simulink model "AUV_MechanicsHullCAD"  (R2020a)
(part 3 of 12)

      mask help: This block creates a flat, single, square tile element. The square tile body is mass-less, so it will not have an effect on the dynamic simulation. This square tile element can be used as a graphic reference by itself, or as part of a composite graphic reference made of an array of interconnected tiles. The square tile is aligned with the XY plane, and the block provides frame connector ports to the middle points on each of the four sides of the body of the square - right (+X), left (-X), top (+Y) and bottom (-Y). All dimensions are in meters.
      settings: PortSchema="{\"entries\":[{\"content\":{\"sides\":[{\"content\":{\"connectorIds\":[\"LConn1\"]},\"type\":\"ConnectorPlacement.EquallySpacedRectSide\",\"uuid\":\"a971723f-ea37-4e9b-910b-501b94fb0ba2\"},{\"content\":{\"connectorIds\":[\"RConn1\"],\"side\":\"RIGHT\"},\"type\":\"ConnectorPlacement.EquallySpacedRectSide\",\"uuid\":\"e50175c1-005c-4b0b-bced-b882197eaab2\"},{\"content\":{\"connectorIds\":[\"LConn2\"],\"side\":\"TOP\"},\"type\":\"ConnectorPlacement.EquallySpacedRectSide\",\"uuid\":\"2a04a964-d53e-47ee-8c79-d53dd599bafe\"},{\"content\":{\"connectorIds\":[\"RConn2\"],\"side\":\"BOTTOM\"},\"type\":\"ConnectorPlacement.EquallySpacedRectSide\",\"uuid\":\"a0066dd6-a193-491c-afbe-bac00dfc3505\"}]},\"type\":\"ConnectorPlacement.EquallySpacedConnector\",\"uuid\":\"c80211c6-bb24-481b-97ca-2752015f3b18\"}],\"packageUris\":[\"http://schema.mathworks.com/mf0/Connector/19700101\"],\"version\":\"1.0\"}"
  Tile83 : Subsystem  mask(Square Tile){side=side, thickness=thick, color=color1, opacity=opacity}
      mask prompts: side "Side (m) :"; thickness "Thickness (m) :"; color "Color [RGB] :"; opacity "Opacity (0...1) :"
      mask help: This block creates a flat, single, square tile element. The square tile body is mass-less, so it will not have an effect on the dynamic simulation. This square tile element can be used as a graphic reference by itself, or as part of a composite graphic reference made of an array of interconnected tiles. The square tile is aligned with the XY plane, and the block provides frame connector ports to the middle points on each of the four sides of the body of the square - right (+X), left (-X), top (+Y) and bottom (-Y). All dimensions are in meters.
      settings: PortSchema="{\"entries\":[{\"content\":{\"sides\":[{\"content\":{\"connectorIds\":[\"LConn1\"]},\"type\":\"ConnectorPlacement.EquallySpacedRectSide\",\"uuid\":\"a971723f-ea37-4e9b-910b-501b94fb0ba2\"},{\"content\":{\"connectorIds\":[\"RConn1\"],\"side\":\"RIGHT\"},\"type\":\"ConnectorPlacement.EquallySpacedRectSide\",\"uuid\":\"e50175c1-005c-4b0b-bced-b882197eaab2\"},{\"content\":{\"connectorIds\":[\"LConn2\"],\"side\":\"TOP\"},\"type\":\"ConnectorPlacement.EquallySpacedRectSide\",\"uuid\":\"2a04a964-d53e-47ee-8c79-d53dd599bafe\"},{\"content\":{\"connectorIds\":[\"RConn2\"],\"side\":\"BOTTOM\"},\"type\":\"ConnectorPlacement.EquallySpacedRectSide\",\"uuid\":\"a0066dd6-a193-491c-afbe-bac00dfc3505\"}]},\"type\":\"ConnectorPlacement.EquallySpacedConnector\",\"uuid\":\"c80211c6-bb24-481b-97ca-2752015f3b18\"}],\"packageUris\":[\"http://schema.mathworks.com/mf0/Connector/19700101\"],\"version\":\"1.0\"}"
  Tile84 : Subsystem  mask(Square Tile){side=side, thickness=thick, color=color1, opacity=opacity}
      mask prompts: side "Side (m) :"; thickness "Thickness (m) :"; color "Color [RGB] :"; opacity "Opacity (0...1) :"
      mask help: This block creates a flat, single, square tile element. The square tile body is mass-less, so it will not have an effect on the dynamic simulation. This square tile element can be used as a graphic reference by itself, or as part of a composite graphic reference made of an array of interconnected tiles. The square tile is aligned with the XY plane, and the block provides frame connector ports to the middle points on each of the four sides of the body of the square - right (+X), left (-X), top (+Y) and bottom (-Y). All dimensions are in meters.
      settings: PortSchema="{\"entries\":[{\"content\":{\"sides\":[{\"content\":{\"connectorIds\":[\"LConn1\"]},\"type\":\"ConnectorPlacement.EquallySpacedRectSide\",\"uuid\":\"a971723f-ea37-4e9b-910b-501b94fb0ba2\"},{\"content\":{\"connectorIds\":[\"RConn1\"],\"side\":\"RIGHT\"},\"type\":\"ConnectorPlacement.EquallySpacedRectSide\",\"uuid\":\"e50175c1-005c-4b0b-bced-b882197eaab2\"},{\"content\":{\"connectorIds\":[\"LConn2\"],\"side\":\"TOP\"},\"type\":\"ConnectorPlacement.EquallySpacedRectSide\",\"uuid\":\"2a04a964-d53e-47ee-8c79-d53dd599bafe\"},{\"content\":{\"connectorIds\":[\"RConn2\"],\"side\":\"BOTTOM\"},\"type\":\"ConnectorPlacement.EquallySpacedRectSide\",\"uuid\":\"a0066dd6-a193-491c-afbe-bac00dfc3505\"}]},\"type\":\"ConnectorPlacement.EquallySpacedConnector\",\"uuid\":\"c80211c6-bb24-481b-97ca-2752015f3b18\"}],\"packageUris\":[\"http://schema.mathworks.com/mf0/Connector/19700101\"],\"version\":\"1.0\"}"
  Tile85 : Subsystem  mask(Square Tile){side=side, thickness=thick, color=color2, opacity=opacity}
      mask prompts: side "Side (m) :"; thickness "Thickness (m) :"; color "Color [RGB] :"; opacity "Opacity (0...1) :"
      mask help: This block creates a flat, single, square tile element. The square tile body is mass-less, so it will not have an effect on the dynamic simulation. This square tile element can be used as a graphic reference by itself, or as part of a composite graphic reference made of an array of interconnected tiles. The square tile is aligned with the XY plane, and the block provides frame connector ports to the middle points on each of the four sides of the body of the square - right (+X), left (-X), top (+Y) and bottom (-Y). All dimensions are in meters.
      settings: PortSchema="{\"entries\":[{\"content\":{\"sides\":[{\"content\":{\"connectorIds\":[\"LConn1\"]},\"type\":\"ConnectorPlacement.EquallySpacedRectSide\",\"uuid\":\"a971723f-ea37-4e9b-910b-501b94fb0ba2\"},{\"content\":{\"connectorIds\":[\"RConn1\"],\"side\":\"RIGHT\"},\"type\":\"ConnectorPlacement.EquallySpacedRectSide\",\"uuid\":\"e50175c1-005c-4b0b-bced-b882197eaab2\"},{\"content\":{\"connectorIds\":[\"LConn2\"],\"side\":\"TOP\"},\"type\":\"ConnectorPlacement.EquallySpacedRectSide\",\"uuid\":\"2a04a964-d53e-47ee-8c79-d53dd599bafe\"},{\"content\":{\"connectorIds\":[\"RConn2\"],\"side\":\"BOTTOM\"},\"type\":\"ConnectorPlacement.EquallySpacedRectSide\",\"uuid\":\"a0066dd6-a193-491c-afbe-bac00dfc3505\"}]},\"type\":\"ConnectorPlacement.EquallySpacedConnector\",\"uuid\":\"c80211c6-bb24-481b-97ca-2752015f3b18\"}],\"packageUris\":[\"http://schema.mathworks.com/mf0/Connector/19700101\"],\"version\":\"1.0\"}"
  Tile86 : Subsystem  mask(Square Tile){side=side, thickness=thick, color=color1, opacity=opacity}
      mask prompts: side "Side (m) :"; thickness "Thickness (m) :"; color "Color [RGB] :"; opacity "Opacity (0...1) :"
      mask help: This block creates a flat, single, square tile element. The square tile body is mass-less, so it will not have an effect on the dynamic simulation. This square tile element can be used as a graphic reference by itself, or as part of a composite graphic reference made of an array of interconnected tiles. The square tile is aligned with the XY plane, and the block provides frame connector ports to the middle points on each of the four sides of the body of the square - right (+X), left (-X), top (+Y) and bottom (-Y). All dimensions are in meters.
      settings: PortSchema="{\"entries\":[{\"content\":{\"sides\":[{\"content\":{\"connectorIds\":[\"LConn1\"]},\"type\":\"ConnectorPlacement.EquallySpacedRectSide\",\"uuid\":\"a971723f-ea37-4e9b-910b-501b94fb0ba2\"},{\"content\":{\"connectorIds\":[\"RConn1\"],\"side\":\"RIGHT\"},\"type\":\"ConnectorPlacement.EquallySpacedRectSide\",\"uuid\":\"e50175c1-005c-4b0b-bced-b882197eaab2\"},{\"content\":{\"connectorIds\":[\"LConn2\"],\"side\":\"TOP\"},\"type\":\"ConnectorPlacement.EquallySpacedRectSide\",\"uuid\":\"2a04a964-d53e-47ee-8c79-d53dd599bafe\"},{\"content\":{\"connectorIds\":[\"RConn2\"],\"side\":\"BOTTOM\"},\"type\":\"ConnectorPlacement.EquallySpacedRectSide\",\"uuid\":\"a0066dd6-a193-491c-afbe-bac00dfc3505\"}]},\"type\":\"ConnectorPlacement.EquallySpacedConnector\",\"uuid\":\"c80211c6-bb24-481b-97ca-2752015f3b18\"}],\"packageUris\":[\"http://schema.mathworks.com/mf0/Connector/19700101\"],\"version\":\"1.0\"}"
  Tile87 : Subsystem  mask(Square Tile){side=side, thickness=thick, color=color2, opacity=opacity}
      mask prompts: side "Side (m) :"; thickness "Thickness (m) :"; color "Color [RGB] :"; opacity "Opacity (0...1) :"
      mask help: This block creates a flat, single, square tile element. The square tile body is mass-less, so it will not have an effect on the dynamic simulation. This square tile element can be used as a graphic reference by itself, or as part of a composite graphic reference made of an array of interconnected tiles. The square tile is aligned with the XY plane, and the block provides frame connector ports to the middle points on each of the four sides of the body of the square - right (+X), left (-X), top (+Y) and bottom (-Y). All dimensions are in meters.
      settings: PortSchema="{\"entries\":[{\"content\":{\"sides\":[{\"content\":{\"connectorIds\":[\"LConn1\"]},\"type\":\"ConnectorPlacement.EquallySpacedRectSide\",\"uuid\":\"a971723f-ea37-4e9b-910b-501b94fb0ba2\"},{\"content\":{\"connectorIds\":[\"RConn1\"],\"side\":\"RIGHT\"},\"type\":\"ConnectorPlacement.EquallySpacedRectSide\",\"uuid\":\"e50175c1-005c-4b0b-bced-b882197eaab2\"},{\"content\":{\"connectorIds\":[\"LConn2\"],\"side\":\"TOP\"},\"type\":\"ConnectorPlacement.EquallySpacedRectSide\",\"uuid\":\"2a04a964-d53e-47ee-8c79-d53dd599bafe\"},{\"content\":{\"connectorIds\":[\"RConn2\"],\"side\":\"BOTTOM\"},\"type\":\"ConnectorPlacement.EquallySpacedRectSide\",\"uuid\":\"a0066dd6-a193-491c-afbe-bac00dfc3505\"}]},\"type\":\"ConnectorPlacement.EquallySpacedConnector\",\"uuid\":\"c80211c6-bb24-481b-97ca-2752015f3b18\"}],\"packageUris\":[\"http://schema.mathworks.com/mf0/Connector/19700101\"],\"version\":\"1.0\"}"
  Tile88 : Subsystem  mask(Square Tile){side=side, thickness=thick, color=color1, opacity=opacity}
      mask prompts: side "Side (m) :"; thickness "Thickness (m) :"; color "Color [RGB] :"; opacity "Opacity (0...1) :"
      mask help: This block creates a flat, single, square tile element. The square tile body is mass-less, so it will not have an effect on the dynamic simulation. This square tile element can be used as a graphic reference by itself, or as part of a composite graphic reference made of an array of interconnected tiles. The square tile is aligned with the XY plane, and the block provides frame connector ports to the middle points on each of the four sides of the body of the square - right (+X), left (-X), top (+Y) and bottom (-Y). All dimensions are in meters.
      settings: PortSchema="{\"entries\":[{\"content\":{\"sides\":[{\"content\":{\"connectorIds\":[\"LConn1\"]},\"type\":\"ConnectorPlacement.EquallySpacedRectSide\",\"uuid\":\"a971723f-ea37-4e9b-910b-501b94fb0ba2\"},{\"content\":{\"connectorIds\":[\"RConn1\"],\"side\":\"RIGHT\"},\"type\":\"ConnectorPlacement.EquallySpacedRectSide\",\"uuid\":\"e50175c1-005c-4b0b-bced-b882197eaab2\"},{\"content\":{\"connectorIds\":[\"LConn2\"],\"side\":\"TOP\"},\"type\":\"ConnectorPlacement.EquallySpacedRectSide\",\"uuid\":\"2a04a964-d53e-47ee-8c79-d53dd599bafe\"},{\"content\":{\"connectorIds\":[\"RConn2\"],\"side\":\"BOTTOM\"},\"type\":\"ConnectorPlacement.EquallySpacedRectSide\",\"uuid\":\"a0066dd6-a193-491c-afbe-bac00dfc3505\"}]},\"type\":\"ConnectorPlacement.EquallySpacedConnector\",\"uuid\":\"c80211c6-bb24-481b-97ca-2752015f3b18\"}],\"packageUris\":[\"http://schema.mathworks.com/mf0/Connector/19700101\"],\"version\":\"1.0\"}"
  Tile89 : Subsystem  mask(Square Tile){side=side, thickness=thick, color=color2, opacity=opacity}
      mask prompts: side "Side (m) :"; thickness "Thickness (m) :"; color "Color [RGB] :"; opacity "Opacity (0...1) :"
      mask help: This block creates a flat, single, square tile element. The square tile body is mass-less, so it will not have an effect on the dynamic simulation. This square tile element can be used as a graphic reference by itself, or as part of a composite graphic reference made of an array of interconnected tiles. The square tile is aligned with the XY plane, and the block provides frame connector ports to the middle points on each of the four sides of the body of the square - right (+X), left (-X), top (+Y) and bottom (-Y). All dimensions are in meters.
      settings: PortSchema="{\"entries\":[{\"content\":{\"sides\":[{\"content\":{\"connectorIds\":[\"LConn1\"]},\"type\":\"ConnectorPlacement.EquallySpacedRectSide\",\"uuid\":\"a971723f-ea37-4e9b-910b-501b94fb0ba2\"},{\"content\":{\"connectorIds\":[\"RConn1\"],\"side\":\"RIGHT\"},\"type\":\"ConnectorPlacement.EquallySpacedRectSide\",\"uuid\":\"e50175c1-005c-4b0b-bced-b882197eaab2\"},{\"content\":{\"connectorIds\":[\"LConn2\"],\"side\":\"TOP\"},\"type\":\"ConnectorPlacement.EquallySpacedRectSide\",\"uuid\":\"2a04a964-d53e-47ee-8c79-d53dd599bafe\"},{\"content\":{\"connectorIds\":[\"RConn2\"],\"side\":\"BOTTOM\"},\"type\":\"ConnectorPlacement.EquallySpacedRectSide\",\"uuid\":\"a0066dd6-a193-491c-afbe-bac00dfc3505\"}]},\"type\":\"ConnectorPlacement.EquallySpacedConnector\",\"uuid\":\"c80211c6-bb24-481b-97ca-2752015f3b18\"}],\"packageUris\":[\"http://schema.mathworks.com/mf0/Connector/19700101\"],\"version\":\"1.0\"}"
  Tile9 : Subsystem  mask(Square Tile){side=side, thickness=thick, color=color1, opacity=opacity}
      mask prompts: side "Side (m) :"; thickness "Thickness (m) :"; color "Color [RGB] :"; opacity "Opacity (0...1) :"
      mask help: This block creates a flat, single, square tile element. The square tile body is mass-less, so it will not have an effect on the dynamic simulation. This square tile element can be used as a graphic reference by itself, or as part of a composite graphic reference made of an array of interconnected tiles. The square tile is aligned with the XY plane, and the block provides frame connector ports to the middle points on each of the four sides of the body of the square - right (+X), left (-X), top (+Y) and bottom (-Y). All dimensions are in meters.
      settings: PortSchema="{\"entries\":[{\"content\":{\"sides\":[{\"content\":{\"connectorIds\":[\"LConn1\"]},\"type\":\"ConnectorPlacement.EquallySpacedRectSide\",\"uuid\":\"a971723f-ea37-4e9b-910b-501b94fb0ba2\"},{\"content\":{\"connectorIds\":[\"RConn1\"],\"side\":\"RIGHT\"},\"type\":\"ConnectorPlacement.EquallySpacedRectSide\",\"uuid\":\"e50175c1-005c-4b0b-bced-b882197eaab2\"},{\"content\":{\"connectorIds\":[\"LConn2\"],\"side\":\"TOP\"},\"type\":\"ConnectorPlacement.EquallySpacedRectSide\",\"uuid\":\"2a04a964-d53e-47ee-8c79-d53dd599bafe\"},{\"content\":{\"connectorIds\":[\"RConn2\"],\"side\":\"BOTTOM\"},\"type\":\"ConnectorPlacement.EquallySpacedRectSide\",\"uuid\":\"a0066dd6-a193-491c-afbe-bac00dfc3505\"}]},\"type\":\"ConnectorPlacement.EquallySpacedConnector\",\"uuid\":\"c80211c6-bb24-481b-97ca-2752015f3b18\"}],\"packageUris\":[\"http://schema.mathworks.com/mf0/Connector/19700101\"],\"version\":\"1.0\"}"
  Tile90 : Subsystem  mask(Square Tile){side=side, thickness=thick, color=color1, opacity=opacity}
      mask prompts: side "Side (m) :"; thickness "Thickness (m) :"; color "Color [RGB] :"; opacity "Opacity (0...1) :"
      mask help: This block creates a flat, single, square tile element. The square tile body is mass-less, so it will not have an effect on the dynamic simulation. This square tile element can be used as a graphic reference by itself, or as part of a composite graphic reference made of an array of interconnected tiles. The square tile is aligned with the XY plane, and the block provides frame connector ports to the middle points on each of the four sides of the body of the square - right (+X), left (-X), top (+Y) and bottom (-Y). All dimensions are in meters.
      settings: PortSchema="{\"entries\":[{\"content\":{\"sides\":[{\"content\":{\"connectorIds\":[\"LConn1\"]},\"type\":\"ConnectorPlacement.EquallySpacedRectSide\",\"uuid\":\"a971723f-ea37-4e9b-910b-501b94fb0ba2\"},{\"content\":{\"connectorIds\":[\"RConn1\"],\"side\":\"RIGHT\"},\"type\":\"ConnectorPlacement.EquallySpacedRectSide\",\"uuid\":\"e50175c1-005c-4b0b-bced-b882197eaab2\"},{\"content\":{\"connectorIds\":[\"LConn2\"],\"side\":\"TOP\"},\"type\":\"ConnectorPlacement.EquallySpacedRectSide\",\"uuid\":\"2a04a964-d53e-47ee-8c79-d53dd599bafe\"},{\"content\":{\"connectorIds\":[\"RConn2\"],\"side\":\"BOTTOM\"},\"type\":\"ConnectorPlacement.EquallySpacedRectSide\",\"uuid\":\"a0066dd6-a193-491c-afbe-bac00dfc3505\"}]},\"type\":\"ConnectorPlacement.EquallySpacedConnector\",\"uuid\":\"c80211c6-bb24-481b-97ca-2752015f3b18\"}],\"packageUris\":[\"http://schema.mathworks.com/mf0/Connector/19700101\"],\"version\":\"1.0\"}"
  Tile91 : Subsystem  mask(Square Tile){side=side, thickness=thick, color=color1, opacity=opacity}
      mask prompts: side "Side (m) :"; thickness "Thickness (m) :"; color "Color [RGB] :"; opacity "Opacity (0...1) :"
      mask help: This block creates a flat, single, square tile element. The square tile body is mass-less, so it will not have an effect on the dynamic simulation. This square tile element can be used as a graphic reference by itself, or as part of a composite graphic reference made of an array of interconnected tiles. The square tile is aligned with the XY plane, and the block provides frame connector ports to the middle points on each of the four sides of the body of the square - right (+X), left (-X), top (+Y) and bottom (-Y). All dimensions are in meters.
      settings: PortSchema="{\"entries\":[{\"content\":{\"sides\":[{\"content\":{\"connectorIds\":[\"LConn1\"]},\"type\":\"ConnectorPlacement.EquallySpacedRectSide\",\"uuid\":\"a971723f-ea37-4e9b-910b-501b94fb0ba2\"},{\"content\":{\"connectorIds\":[\"RConn1\"],\"side\":\"RIGHT\"},\"type\":\"ConnectorPlacement.EquallySpacedRectSide\",\"uuid\":\"e50175c1-005c-4b0b-bced-b882197eaab2\"},{\"content\":{\"connectorIds\":[\"LConn2\"],\"side\":\"TOP\"},\"type\":\"ConnectorPlacement.EquallySpacedRectSide\",\"uuid\":\"2a04a964-d53e-47ee-8c79-d53dd599bafe\"},{\"content\":{\"connectorIds\":[\"RConn2\"],\"side\":\"BOTTOM\"},\"type\":\"ConnectorPlacement.EquallySpacedRectSide\",\"uuid\":\"a0066dd6-a193-491c-afbe-bac00dfc3505\"}]},\"type\":\"ConnectorPlacement.EquallySpacedConnector\",\"uuid\":\"c80211c6-bb24-481b-97ca-2752015f3b18\"}],\"packageUris\":[\"http://schema.mathworks.com/mf0/Connector/19700101\"],\"version\":\"1.0\"}"
  Tile92 : Subsystem  mask(Square Tile){side=side, thickness=thick, color=color2, opacity=opacity}
      mask prompts: side "Side (m) :"; thickness "Thickness (m) :"; color "Color [RGB] :"; opacity "Opacity (0...1) :"
      mask help: This block creates a flat, single, square tile element. The square tile body is mass-less, so it will not have an effect on the dynamic simulation. This square tile element can be used as a graphic reference by itself, or as part of a composite graphic reference made of an array of interconnected tiles. The square tile is aligned with the XY plane, and the block provides frame connector ports to the middle points on each of the four sides of the body of the square - right (+X), left (-X), top (+Y) and bottom (-Y). All dimensions are in meters.
      settings: PortSchema="{\"entries\":[{\"content\":{\"sides\":[{\"content\":{\"connectorIds\":[\"LConn1\"]},\"type\":\"ConnectorPlacement.EquallySpacedRectSide\",\"uuid\":\"a971723f-ea37-4e9b-910b-501b94fb0ba2\"},{\"content\":{\"connectorIds\":[\"RConn1\"],\"side\":\"RIGHT\"},\"type\":\"ConnectorPlacement.EquallySpacedRectSide\",\"uuid\":\"e50175c1-005c-4b0b-bced-b882197eaab2\"},{\"content\":{\"connectorIds\":[\"LConn2\"],\"side\":\"TOP\"},\"type\":\"ConnectorPlacement.EquallySpacedRectSide\",\"uuid\":\"2a04a964-d53e-47ee-8c79-d53dd599bafe\"},{\"content\":{\"connectorIds\":[\"RConn2\"],\"side\":\"BOTTOM\"},\"type\":\"ConnectorPlacement.EquallySpacedRectSide\",\"uuid\":\"a0066dd6-a193-491c-afbe-bac00dfc3505\"}]},\"type\":\"ConnectorPlacement.EquallySpacedConnector\",\"uuid\":\"c80211c6-bb24-481b-97ca-2752015f3b18\"}],\"packageUris\":[\"http://schema.mathworks.com/mf0/Connector/19700101\"],\"version\":\"1.0\"}"
  Tile93 : Subsystem  mask(Square Tile){side=side, thickness=thick, color=color2, opacity=opacity}
      mask prompts: side "Side (m) :"; thickness "Thickness (m) :"; color "Color [RGB] :"; opacity "Opacity (0...1) :"
      mask help: This block creates a flat, single, square tile element. The square tile body is mass-less, so it will not have an effect on the dynamic simulation. This square tile element can be used as a graphic reference by itself, or as part of a composite graphic reference made of an array of interconnected tiles. The square tile is aligned with the XY plane, and the block provides frame connector ports to the middle points on each of the four sides of the body of the square - right (+X), left (-X), top (+Y) and bottom (-Y). All dimensions are in meters.
      settings: PortSchema="{\"entries\":[{\"content\":{\"sides\":[{\"content\":{\"connectorIds\":[\"LConn1\"]},\"type\":\"ConnectorPlacement.EquallySpacedRectSide\",\"uuid\":\"a971723f-ea37-4e9b-910b-501b94fb0ba2\"},{\"content\":{\"connectorIds\":[\"RConn1\"],\"side\":\"RIGHT\"},\"type\":\"ConnectorPlacement.EquallySpacedRectSide\",\"uuid\":\"e50175c1-005c-4b0b-bced-b882197eaab2\"},{\"content\":{\"connectorIds\":[\"LConn2\"],\"side\":\"TOP\"},\"type\":\"ConnectorPlacement.EquallySpacedRectSide\",\"uuid\":\"2a04a964-d53e-47ee-8c79-d53dd599bafe\"},{\"content\":{\"connectorIds\":[\"RConn2\"],\"side\":\"BOTTOM\"},\"type\":\"ConnectorPlacement.EquallySpacedRectSide\",\"uuid\":\"a0066dd6-a193-491c-afbe-bac00dfc3505\"}]},\"type\":\"ConnectorPlacement.EquallySpacedConnector\",\"uuid\":\"c80211c6-bb24-481b-97ca-2752015f3b18\"}],\"packageUris\":[\"http://schema.mathworks.com/mf0/Connector/19700101\"],\"version\":\"1.0\"}"
  Tile94 : Subsystem  mask(Square Tile){side=side, thickness=thick, color=color1, opacity=opacity}
      mask prompts: side "Side (m) :"; thickness "Thickness (m) :"; color "Color [RGB] :"; opacity "Opacity (0...1) :"
      mask help: This block creates a flat, single, square tile element. The square tile body is mass-less, so it will not have an effect on the dynamic simulation. This square tile element can be used as a graphic reference by itself, or as part of a composite graphic reference made of an array of interconnected tiles. The square tile is aligned with the XY plane, and the block provides frame connector ports to the middle points on each of the four sides of the body of the square - right (+X), left (-X), top (+Y) and bottom (-Y). All dimensions are in meters.
      settings: PortSchema="{\"entries\":[{\"content\":{\"sides\":[{\"content\":{\"connectorIds\":[\"LConn1\"]},\"type\":\"ConnectorPlacement.EquallySpacedRectSide\",\"uuid\":\"a971723f-ea37-4e9b-910b-501b94fb0ba2\"},{\"content\":{\"connectorIds\":[\"RConn1\"],\"side\":\"RIGHT\"},\"type\":\"ConnectorPlacement.EquallySpacedRectSide\",\"uuid\":\"e50175c1-005c-4b0b-bced-b882197eaab2\"},{\"content\":{\"connectorIds\":[\"LConn2\"],\"side\":\"TOP\"},\"type\":\"ConnectorPlacement.EquallySpacedRectSide\",\"uuid\":\"2a04a964-d53e-47ee-8c79-d53dd599bafe\"},{\"content\":{\"connectorIds\":[\"RConn2\"],\"side\":\"BOTTOM\"},\"type\":\"ConnectorPlacement.EquallySpacedRectSide\",\"uuid\":\"a0066dd6-a193-491c-afbe-bac00dfc3505\"}]},\"type\":\"ConnectorPlacement.EquallySpacedConnector\",\"uuid\":\"c80211c6-bb24-481b-97ca-2752015f3b18\"}],\"packageUris\":[\"http://schema.mathworks.com/mf0/Connector/19700101\"],\"version\":\"1.0\"}"
  Tile95 : Subsystem  mask(Square Tile){side=side, thickness=thick, color=color2, opacity=opacity}
      mask prompts: side "Side (m) :"; thickness "Thickness (m) :"; color "Color [RGB] :"; opacity "Opacity (0...1) :"
      mask help: This block creates a flat, single, square tile element. The square tile body is mass-less, so it will not have an effect on the dynamic simulation. This square tile element can be used as a graphic reference by itself, or as part of a composite graphic reference made of an array of interconnected tiles. The square tile is aligned with the XY plane, and the block provides frame connector ports to the middle points on each of the four sides of the body of the square - right (+X), left (-X), top (+Y) and bottom (-Y). All dimensions are in meters.
      settings: PortSchema="{\"entries\":[{\"content\":{\"sides\":[{\"content\":{\"connectorIds\":[\"LConn1\"]},\"type\":\"ConnectorPlacement.EquallySpacedRectSide\",\"uuid\":\"a971723f-ea37-4e9b-910b-501b94fb0ba2\"},{\"content\":{\"connectorIds\":[\"RConn1\"],\"side\":\"RIGHT\"},\"type\":\"ConnectorPlacement.EquallySpacedRectSide\",\"uuid\":\"e50175c1-005c-4b0b-bced-b882197eaab2\"},{\"content\":{\"connectorIds\":[\"LConn2\"],\"side\":\"TOP\"},\"type\":\"ConnectorPlacement.EquallySpacedRectSide\",\"uuid\":\"2a04a964-d53e-47ee-8c79-d53dd599bafe\"},{\"content\":{\"connectorIds\":[\"RConn2\"],\"side\":\"BOTTOM\"},\"type\":\"ConnectorPlacement.EquallySpacedRectSide\",\"uuid\":\"a0066dd6-a193-491c-afbe-bac00dfc3505\"}]},\"type\":\"ConnectorPlacement.EquallySpacedConnector\",\"uuid\":\"c80211c6-bb24-481b-97ca-2752015f3b18\"}],\"packageUris\":[\"http://schema.mathworks.com/mf0/Connector/19700101\"],\"version\":\"1.0\"}"
  Tile96 : Subsystem  mask(Square Tile){side=side, thickness=thick, color=color1, opacity=opacity}
      mask prompts: side "Side (m) :"; thickness "Thickness (m) :"; color "Color [RGB] :"; opacity "Opacity (0...1) :"
      mask help: This block creates a flat, single, square tile element. The square tile body is mass-less, so it will not have an effect on the dynamic simulation. This square tile element can be used as a graphic reference by itself, or as part of a composite graphic reference made of an array of interconnected tiles. The square tile is aligned with the XY plane, and the block provides frame connector ports to the middle points on each of the four sides of the body of the square - right (+X), left (-X), top (+Y) and bottom (-Y). All dimensions are in meters.
      settings: PortSchema="{\"entries\":[{\"content\":{\"sides\":[{\"content\":{\"connectorIds\":[\"LConn1\"]},\"type\":\"ConnectorPlacement.EquallySpacedRectSide\",\"uuid\":\"a971723f-ea37-4e9b-910b-501b94fb0ba2\"},{\"content\":{\"connectorIds\":[\"RConn1\"],\"side\":\"RIGHT\"},\"type\":\"ConnectorPlacement.EquallySpacedRectSide\",\"uuid\":\"e50175c1-005c-4b0b-bced-b882197eaab2\"},{\"content\":{\"connectorIds\":[\"LConn2\"],\"side\":\"TOP\"},\"type\":\"ConnectorPlacement.EquallySpacedRectSide\",\"uuid\":\"2a04a964-d53e-47ee-8c79-d53dd599bafe\"},{\"content\":{\"connectorIds\":[\"RConn2\"],\"side\":\"BOTTOM\"},\"type\":\"ConnectorPlacement.EquallySpacedRectSide\",\"uuid\":\"a0066dd6-a193-491c-afbe-bac00dfc3505\"}]},\"type\":\"ConnectorPlacement.EquallySpacedConnector\",\"uuid\":\"c80211c6-bb24-481b-97ca-2752015f3b18\"}],\"packageUris\":[\"http://schema.mathworks.com/mf0/Connector/19700101\"],\"version\":\"1.0\"}"
  Tile97 : Subsystem  mask(Square Tile){side=side, thickness=thick, color=color2, opacity=opacity}
      mask prompts: side "Side (m) :"; thickness "Thickness (m) :"; color "Color [RGB] :"; opacity "Opacity (0...1) :"
      mask help: This block creates a flat, single, square tile element. The square tile body is mass-less, so it will not have an effect on the dynamic simulation. This square tile element can be used as a graphic reference by itself, or as part of a composite graphic reference made of an array of interconnected tiles. The square tile is aligned with the XY plane, and the block provides frame connector ports to the middle points on each of the four sides of the body of the square - right (+X), left (-X), top (+Y) and bottom (-Y). All dimensions are in meters.
      settings: PortSchema="{\"entries\":[{\"content\":{\"sides\":[{\"content\":{\"connectorIds\":[\"LConn1\"]},\"type\":\"ConnectorPlacement.EquallySpacedRectSide\",\"uuid\":\"a971723f-ea37-4e9b-910b-501b94fb0ba2\"},{\"content\":{\"connectorIds\":[\"RConn1\"],\"side\":\"RIGHT\"},\"type\":\"ConnectorPlacement.EquallySpacedRectSide\",\"uuid\":\"e50175c1-005c-4b0b-bced-b882197eaab2\"},{\"content\":{\"connectorIds\":[\"LConn2\"],\"side\":\"TOP\"},\"type\":\"ConnectorPlacement.EquallySpacedRectSide\",\"uuid\":\"2a04a964-d53e-47ee-8c79-d53dd599bafe\"},{\"content\":{\"connectorIds\":[\"RConn2\"],\"side\":\"BOTTOM\"},\"type\":\"ConnectorPlacement.EquallySpacedRectSide\",\"uuid\":\"a0066dd6-a193-491c-afbe-bac00dfc3505\"}]},\"type\":\"ConnectorPlacement.EquallySpacedConnector\",\"uuid\":\"c80211c6-bb24-481b-97ca-2752015f3b18\"}],\"packageUris\":[\"http://schema.mathworks.com/mf0/Connector/19700101\"],\"version\":\"1.0\"}"
  Tile98 : Subsystem  mask(Square Tile){side=side, thickness=thick, color=color1, opacity=opacity}
      mask prompts: side "Side (m) :"; thickness "Thickness (m) :"; color "Color [RGB] :"; opacity "Opacity (0...1) :"
      mask help: This block creates a flat, single, square tile element. The square tile body is mass-less, so it will not have an effect on the dynamic simulation. This square tile element can be used as a graphic reference by itself, or as part of a composite graphic reference made of an array of interconnected tiles. The square tile is aligned with the XY plane, and the block provides frame connector ports to the middle points on each of the four sides of the body of the square - right (+X), left (-X), top (+Y) and bottom (-Y). All dimensions are in meters.
      settings: PortSchema="{\"entries\":[{\"content\":{\"sides\":[{\"content\":{\"connectorIds\":[\"LConn1\"]},\"type\":\"ConnectorPlacement.EquallySpacedRectSide\",\"uuid\":\"a971723f-ea37-4e9b-910b-501b94fb0ba2\"},{\"content\":{\"connectorIds\":[\"RConn1\"],\"side\":\"RIGHT\"},\"type\":\"ConnectorPlacement.EquallySpacedRectSide\",\"uuid\":\"e50175c1-005c-4b0b-bced-b882197eaab2\"},{\"content\":{\"connectorIds\":[\"LConn2\"],\"side\":\"TOP\"},\"type\":\"ConnectorPlacement.EquallySpacedRectSide\",\"uuid\":\"2a04a964-d53e-47ee-8c79-d53dd599bafe\"},{\"content\":{\"connectorIds\":[\"RConn2\"],\"side\":\"BOTTOM\"},\"type\":\"ConnectorPlacement.EquallySpacedRectSide\",\"uuid\":\"a0066dd6-a193-491c-afbe-bac00dfc3505\"}]},\"type\":\"ConnectorPlacement.EquallySpacedConnector\",\"uuid\":\"c80211c6-bb24-481b-97ca-2752015f3b18\"}],\"packageUris\":[\"http://schema.mathworks.com/mf0/Connector/19700101\"],\"version\":\"1.0\"}"
  Tile99 : Subsystem  mask(Square Tile){side=side, thickness=thick, color=color2, opacity=opacity}
      mask prompts: side "Side (m) :"; thickness "Thickness (m) :"; color "Color [RGB] :"; opacity "Opacity (0...1) :"
      mask help: This block creates a flat, single, square tile element. The square tile body is mass-less, so it will not have an effect on the dynamic simulation. This square tile element can be used as a graphic reference by itself, or as part of a composite graphic reference made of an array of interconnected tiles. The square tile is aligned with the XY plane, and the block provides frame connector ports to the middle points on each of the four sides of the body of the square - right (+X), left (-X), top (+Y) and bottom (-Y). All dimensions are in meters.
      settings: PortSchema="{\"entries\":[{\"content\":{\"sides\":[{\"content\":{\"connectorIds\":[\"LConn1\"]},\"type\":\"ConnectorPlacement.EquallySpacedRectSide\",\"uuid\":\"a971723f-ea37-4e9b-910b-501b94fb0ba2\"},{\"content\":{\"connectorIds\":[\"RConn1\"],\"side\":\"RIGHT\"},\"type\":\"ConnectorPlacement.EquallySpacedRectSide\",\"uuid\":\"e50175c1-005c-4b0b-bced-b882197eaab2\"},{\"content\":{\"connectorIds\":[\"LConn2\"],\"side\":\"TOP\"},\"type\":\"ConnectorPlacement.EquallySpacedRectSide\",\"uuid\":\"2a04a964-d53e-47ee-8c79-d53dd599bafe\"},{\"content\":{\"connectorIds\":[\"RConn2\"],\"side\":\"BOTTOM\"},\"type\":\"ConnectorPlacement.EquallySpacedRectSide\",\"uuid\":\"a0066dd6-a193-491c-afbe-bac00dfc3505\"}]},\"type\":\"ConnectorPlacement.EquallySpacedConnector\",\"uuid\":\"c80211c6-bb24-481b-97ca-2752015f3b18\"}],\"packageUris\":[\"http://schema.mathworks.com/mf0/Connector/19700101\"],\"version\":\"1.0\"}"
  F : PMIOPort  Side=Left
  connections:
  F/RConn1 -- Tile1/LConn1
  Tile2/LConn1 -- Tile1/RConn1
  Tile4/LConn1 -- Tile3/RConn1
  Tile2/RConn1 -- Tile3/LConn1
  Tile6/RConn1 -- Tile7/LConn1
  Tile8/LConn1 -- Tile7/RConn1
  Tile6/LConn1 -- Tile5/RConn1
  Tile5/LConn1 -- Tile4/RConn1
  Tile10/LConn1 -- Tile9/RConn1
  Tile9/LConn1 -- Tile8/RConn1
  Tile15/LConn1 -- Tile14/RConn1
  Tile16/LConn1 -- Tile15/RConn1
  Tile16/RConn1 -- Tile17/LConn1
  Tile18/LConn1 -- Tile17/RConn1
  Tile11/LConn1 -- Tile19/RConn1
  Tile19/LConn1 -- Tile18/RConn1
  Tile12/RConn1 -- Tile13/LConn1
  Tile14/LConn1 -- Tile13/RConn1
  Tile12/LConn2 -- Tile1/RConn2
  Tile20/LConn1 -- Tile11/RConn1
  Tile24/LConn2 -- Tile21/RConn2
  Tile26/LConn1 -- Tile25/RConn1
  Tile24/RConn1 -- Tile25/LConn1
  Tile31/LConn1 -- Tile30/RConn1
  Tile30/LConn1 -- Tile29/RConn1
  Tile23/LConn1 -- Tile31/RConn1
  Tile28/RConn1 -- Tile29/LConn1
  Tile28/LConn1 -- Tile27/RConn1
  Tile27/LConn1 -- Tile26/RConn1
  Tile36/LConn1 -- Tile35/RConn1
  Tile37/LConn1 -- Tile36/RConn1
  Tile22/LConn1 -- Tile40/RConn1
  Tile37/RConn1 -- Tile38/LConn1
  Tile40/LConn1 -- Tile39/RConn1
  Tile39/LConn1 -- Tile38/RConn1
  Tile32/RConn1 -- Tile34/LConn1
  Tile35/LConn1 -- Tile34/RConn1
  Tile32/LConn1 -- Tile21/RConn1
  Tile33/LConn1 -- Tile23/RConn1
  Tile21/LConn2 -- Tile12/RConn2
  Tile43/LConn1 -- Tile41/RConn1
  Tile43/RConn1 -- Tile44/LConn1
  Tile49/LConn1 -- Tile48/RConn1
  Tile50/LConn1 -- Tile49/RConn1
  Tile42/LConn1 -- Tile50/RConn1
  Tile47/RConn1 -- Tile48/LConn1
  Tile47/LConn1 -- Tile46/RConn1
  Tile46/LConn1 -- Tile45/RConn1
  Tile45/LConn1 -- Tile44/RConn1
  Tile41/LConn2 -- Tile24/RConn2
  Tile55/LConn1 -- Tile54/RConn1
  Tile56/LConn1 -- Tile55/RConn1
  Tile56/RConn1 -- Tile57/LConn1
  Tile58/LConn1 -- Tile57/RConn1
  Tile52/RConn1 -- Tile53/LConn1
  Tile51/LConn1 -- Tile59/RConn1
  Tile60/LConn1 -- Tile51/RConn1
  Tile54/LConn1 -- Tile53/RConn1
  Tile59/LConn1 -- Tile58/RConn1
  Tile52/LConn2 -- Tile41/RConn2
  Tile109/LConn1 -- Tile108/RConn1
  Tile110/LConn1 -- Tile101/RConn1
  Tile91/LConn2 -- Tile74/RConn2
  Tile95/LConn1 -- Tile94/RConn1
  Tile97/RConn1 -- Tile98/LConn1
  Tile108/LConn1 -- Tile107/RConn1
  Tile100/LConn1 -- Tile99/RConn1
  Tile99/LConn1 -- Tile98/RConn1
  Tile93/RConn1 -- Tile94/LConn1
  Tile85/LConn1 -- Tile84/RConn1
  Tile89/LConn1 -- Tile88/RConn1
  Tile93/LConn1 -- Tile91/RConn1
  Tile90/LConn1 -- Tile89/RConn1
  Tile87/RConn1 -- Tile88/LConn1
  Tile72/LConn1 -- Tile90/RConn1
  Tile96/LConn1 -- Tile95/RConn1
  Tile87/LConn1 -- Tile86/RConn1
  Tile105/LConn1 -- Tile104/RConn1
  Tile86/LConn1 -- Tile85/RConn1
  Tile77/LConn1 -- Tile76/RConn1
  Tile78/LConn1 -- Tile77/RConn1
  Tile82/RConn1 -- Tile84/LConn1
  Tile78/RConn1 -- Tile79/LConn1
  Tile73/LConn1 -- Tile81/RConn1
  Tile80/LConn1 -- Tile79/RConn1
  Tile81/LConn1 -- Tile80/RConn1
  Tile76/LConn1 -- Tile75/RConn1
  Tile74/LConn2 -- Tile71/RConn2
  Tile92/LConn1 -- Tile100/RConn1
  Tile104/LConn1 -- Tile103/RConn1
  Tile102/LConn2 -- Tile91/RConn2
  Tile83/LConn1 -- Tile73/RConn1
  Tile106/RConn1 -- Tile107/LConn1
  Tile74/RConn1 -- Tile75/LConn1
  Tile97/LConn1 -- Tile96/RConn1
  Tile106/LConn1 -- Tile105/RConn1
  Tile101/LConn1 -- Tile109/RConn1
  Tile82/LConn1 -- Tile71/RConn1
  Tile102/RConn1 -- Tile103/LConn1
  Tile1/LConn2 -- Tile102/RConn2
